simulink model "ECE_431_Homework_5_2"  (R2017a)
settings: Solver=ode23tb  StartTime=0.0  StopTime=.5  MaxStep=1e-4  RelTol=1e-3
libraries: powerlib x20, simulink x1
settings Model: Creator=Kenzie Brian  LastModifiedBy=Kenzie Brian

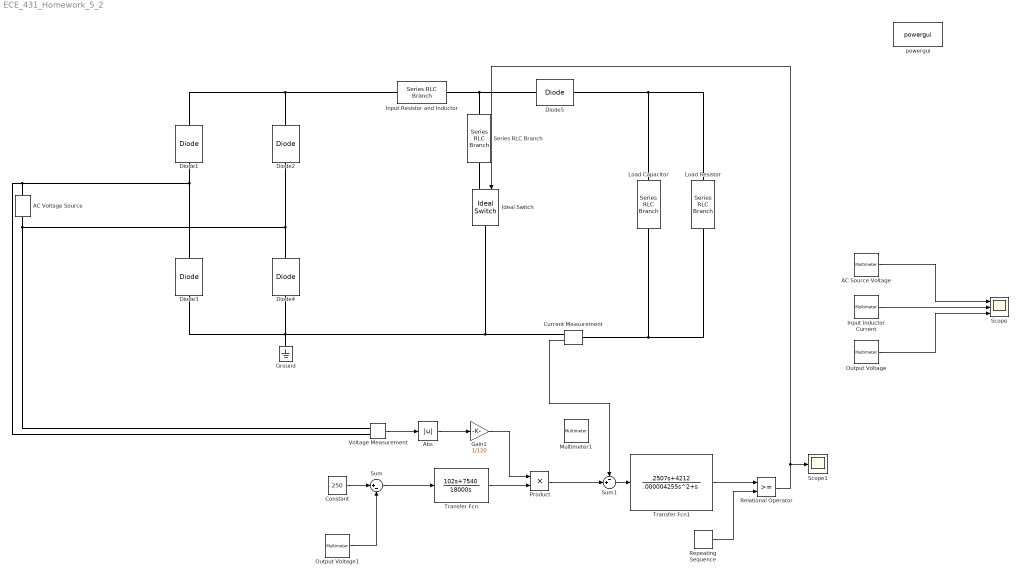
== system ECE_431_Homework_5_2 ==
  AC Source Voltage : powerlib/Measurements/Multimeter  PhasorSimulation=off  OutputType=Complex  sel=2  L=3  Gain=1  yselected={'Usrc: AC Voltage Source'};  PSBOutputType=1  PSBequivalent=0  AxesSetting=[0,0.1,-100,100]  Display=0  SavedBlockNames=-11
  AC Voltage Source : powerlib/Electrical Sources/AC Voltage Source  Amplitude=120  Phase=0  Frequency=60  SampleTime=0  Measurements=Voltage  BusType=swing  Pref=10e3  Qref=0  Qmin=-inf  Qmax=+inf
  Abs : Abs
  Constant : Constant  Value=250
  Current Measurement : powerlib/Measurements/Current Measurement  PhasorSimulation=off  OutputType=Complex  PSBequivalent=0
  Diode{1..5} (5 alike) : powerlib/Power Electronics/Diode  Ron=0.001  Lon=0  Vf=0  IC=0  UseSnubber=0  Rs=500  Cs=250e-9  Measurements=off
  Gain1 : Gain  Gain=1/120
  Ground : powerlib/Elements/Ground  LConnTagsString=a
  Ideal Switch : powerlib/Power Electronics/Ideal Switch  Ron=0.001  Lon=0  IC=0  Rs=1e5  Cs=inf  Measurements=off
  Input Inductor Current : powerlib/Measurements/Multimeter  PhasorSimulation=off  OutputType=Complex  sel=3  L=3  Gain=1  yselected={'Ib: Input Resistor and Inductor'};  PSBOutputType=1  PSBequivalent=0  AxesSetting=[0,0.1,-100,100]  Display=0  SavedBlockNames=-11
  Input Resistor and Inductor : powerlib/Elements/Series RLC Branch  LConnTagsString=__new0  RConnTagsString=__new0  BranchType=RL  Resistance=0  Inductance=1e-3  SetiL0=off  InitialCurrent=0  Capacitance=1e-6  Setx0=off  InitialVoltage=0  Measurements=Branch current
  Load Resistor : powerlib/Elements/Series RLC Branch  LConnTagsString=__new0  RConnTagsString=__new0  BranchType=R  Resistance=250  Inductance=1e-3  SetiL0=off  InitialCurrent=0  Capacitance=1e-6  Setx0=off  InitialVoltage=0  Measurements=Branch voltage
  Load Capacitor : powerlib/Elements/Series RLC Branch  LConnTagsString=__new0  RConnTagsString=__new0  BranchType=RC  Resistance=100e-3  Inductance=1e-3  SetiL0=off  InitialCurrent=0  Capacitance=220e-6  Setx0=off  InitialVoltage=0  Measurements=None
  Multimeter1 : powerlib/Measurements/Multimeter  PhasorSimulation=off  OutputType=Complex  sel=[2 1]  L=3  Gain=[1 1]  yselected={'Usrc: AC Voltage Source','Ub: Load Resistor'};  PSBOutputType=1  PSBequivalent=0  AxesSetting=[0,0.1,-100,100]  Display=1  SavedBlockNames=-11
  Output Voltage : powerlib/Measurements/Multimeter  PhasorSimulation=off  OutputType=Complex  sel=1  L=3  Gain=1  yselected={'Ub: Load Resistor'};  PSBOutputType=1  PSBequivalent=0  AxesSetting=[0,0.1,-100,100]  Display=0  SavedBlockNames=-11
  Output Voltage1 : powerlib/Measurements/Multimeter  PhasorSimulation=off  OutputType=Complex  sel=1  L=3  Gain=1  yselected={'Ub: Load Resistor'};  PSBOutputType=1  PSBequivalent=0  AxesSetting=[0,0.1,-100,100]  Display=0  SavedBlockNames=-11
  Product : Product
  Relational Operator : RelationalOperator  OutDataTypeStr=boolean  ZeroCross=off  RndMeth=Simplest
  Repeating Sequence : simulink/Sources/Repeating Sequence  rep_seq_t=[0 1]*10e-6  rep_seq_y=[0 1]
  Scope : Scope  NumInputPorts=3
  Scope1 : Scope
  Series RLC Branch : powerlib/Elements/Series RLC Branch  LConnTagsString=__new0  RConnTagsString=__new0  BranchType=R  Resistance=2  Inductance=1e-3  SetiL0=off  InitialCurrent=0  Capacitance=1e-6  Setx0=off  InitialVoltage=0  Measurements=None
  Sum : Sum  Inputs=|+-
  Sum1 : Sum  Inputs=-+|
  Transfer Fcn : TransferFcn  Numerator=[102 7540]  Denominator=[18000 0]
  Transfer Fcn1 : TransferFcn  Numerator=[.2507 4212]  Denominator=[.000004255 1 0]
  Voltage Measurement : powerlib/Measurements/Voltage Measurement  PhasorSimulation=off  OutputType=Complex  PSBequivalent=0
  powergui : powerlib/powergui  Priority=1  SimulationMode=Continuous  SampleTime=50e-6  frequency=60  Iterations=50  frequencyindice=60  Pbase=100e6  ErrMax=1e-4  UnitsV=kV  UnitsW=MW  buscounter=0  FunctionMessages=off  echomessages=off  EnableUseOfTLC=off  CurrentSourceSwitches=off  DisableSnubberDevices=off  DisableRonSwitches=off  DisableVfSwitches=off  DisplayEquations=off  SolverType=Tustin/Backward Euler (TBE)  Interpol=off  ExternalGateDelay=off  methode=off  Ts=100  x0status=blocks  SPID=on  SwTol=0  HookPort=off  RestoreLinks=warning  ResistiveCurrentMeasurement=off  Frange=[0:2:500]  Ylog=off  Xlog=on  ShowGrid=off  save=off  variable=ZData  structure=0  ZoomFFT=off  StartTime=0.0  cycles=1  DisplayStyle=1  fundamental=60  FreqAxis=off  MaxFrequency=1000  frequencyindicesteady=1  RmsSteady=1  display=off
  wires:
  AC Source Voltage/1 -> Scope/1
  Input Inductor Current/1 -> Scope/2
  Output Voltage/1 -> Scope/3
  Transfer Fcn1/1 -> Relational Operator/1
  Sum1/1 -> Transfer Fcn1/1
  Sum/1 -> Transfer Fcn/1
  Transfer Fcn/1 -> Product/2
  Product/1 -> Sum1/2
  Output Voltage1/1 -> Sum/2
  Constant/1 -> Sum/1
  Voltage Measurement/1 -> Abs/1
  Repeating Sequence/1 -> Relational Operator/2
  Relational Operator/1 -> Scope1/1, Ideal Switch/1
  Abs/1 -> Gain1/1
  Gain1/1 -> Product/1
  Current Measurement/1 -> Sum1/1
  connections:
  Diode4/RConn1 -- Voltage Measurement/LConn1 -- AC Voltage Source/LConn1 -- Diode2/LConn1
  Diode3/RConn1 -- AC Voltage Source/RConn1 -- Voltage Measurement/LConn2 -- Diode1/LConn1
  Diode1/RConn1 -- Input Resistor and Inductor/LConn1 -- Diode2/RConn1
  Diode3/LConn1 -- Ground/LConn1 -- Current Measurement/RConn1 -- Ideal Switch/RConn1 -- Diode4/LConn1
  Load Resistor/LConn1 -- Load Capacitor/LConn1 -- Diode5/RConn1
  Diode5/LConn1 -- Series RLC Branch/LConn1 -- Input Resistor and Inductor/RConn1
  Ideal Switch/LConn1 -- Series RLC Branch/RConn1
  Load Capacitor/RConn1 -- Load Resistor/RConn1 -- Current Measurement/LConn1
